simulink model "ex2"  (R2021b)
settings: Solver=VariableStepAuto  StartTime=0.0  StopTime=10.0  RelTol=1e-3
values from neighbouring files (symbols this model uses):
  A = [-1 0 0; -1 -2 -101; 1 1 0]    [ex1.m]
  Ad = double(Ad)    [ex1.m]
  B = [0 1; 1 -1; 0 0]    [ex1.m]
  Bd = double(Bd)    [ex1.m]
  C = [1 0 101]    [ex1.m]
  Cd = C    [ex1.m]
  D = [0 0]    [ex1.m]
  Dd = D    [ex1.m]
  h = 0.01    [ex1.m]
  ut = [1; -2]    [ex1.m]
undefined symbols (not defined in the file or in its folder): den1z, den2z, num1z, num2z
settings Model: Creator=ananagirlea  LastModifiedBy=ananagirlea

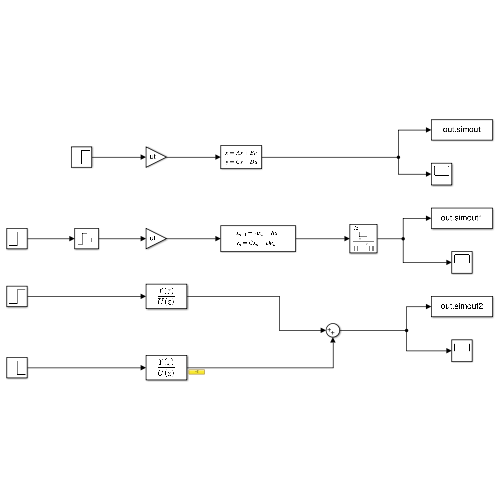
[thumbnail: Simulink's stored preview of the top-level diagram]
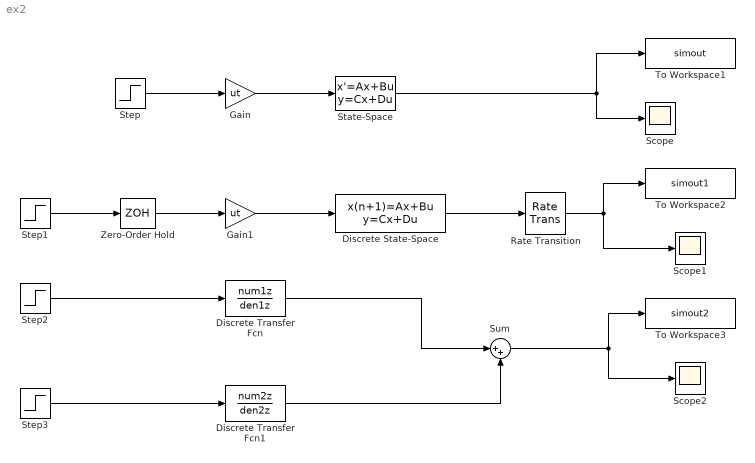
== system ex2 ==
  Discrete Transfer Fcn : DiscreteTransferFcn  Numerator=num1z  Denominator=den1z  SampleTime=h
  Discrete Transfer Fcn1 : DiscreteTransferFcn  Numerator=num2z  Denominator=den2z  SampleTime=h
  Discrete State-Space : DiscreteStateSpace  A=Ad  B=Bd  C=Cd  D=Dd  SampleTime=h
  Gain : Gain  Gain=ut
  Gain1 : Gain  Gain=ut
  Rate Transition : RateTransition
  Scope : Scope
  Scope1 : Scope
  Scope2 : Scope
  State-Space : StateSpace  A=A  B=B  C=C  D=D  InitialCondition=0
  Step : Step  Time=0  SampleTime=0
  Step1 : Step  Time=0  SampleTime=0
  Step2 : Step  Time=0  SampleTime=0
  Step3 : Step  After=-2  SampleTime=0
  Sum : Sum  Inputs=|++
  To Workspace1 : ToWorkspace  VariableName=simout  SaveFormat=Timeseries  SampleTime=-1
  To Workspace2 : ToWorkspace  VariableName=simout1  SaveFormat=Timeseries  SampleTime=-1
  To Workspace3 : ToWorkspace  VariableName=simout2  SaveFormat=Timeseries  SampleTime=-1
  Zero-Order Hold : ZeroOrderHold  SampleTime=h
  wires:
  State-Space/1 -> To Workspace1/1, Scope/1
  Gain/1 -> State-Space/1
  Rate Transition/1 -> To Workspace2/1, Scope1/1
  Step/1 -> Gain/1
  Gain1/1 -> Discrete State-Space/1
  Zero-Order Hold/1 -> Gain1/1
  Step1/1 -> Zero-Order Hold/1
  Discrete State-Space/1 -> Rate Transition/1
  Discrete Transfer Fcn/1 -> Sum/1
  Discrete Transfer Fcn1/1 -> Sum/2
  Sum/1 -> To Workspace3/1, Scope2/1
  Step2/1 -> Discrete Transfer Fcn/1
  Step3/1 -> Discrete Transfer Fcn1/1
